simulink subsystem "VehicleBody6DOFSSC"  (R2024a)
settings: Solver=VariableStepAuto  StartTime=0.0  StopTime=10.0  RelTol=1e-3
undefined symbols (not defined in the file): BdyFrm, EnvAirDen, InertFrm, PlntVehAeroDragCff, PlntVehAeroFrntArea, PlntVehAeroLiftCff, PlntVehCGHgtAxl, PlntVehDstCGFrntAxl, PlntVehDstCGRearAxl, PlntVehInitLatPos, PlntVehInitVertPos, PlntVehMass, PlntVehMultiBody, PlntVehPitchMomentInertia, PlntVehRollMomentInertia, PlntVehYawMomentInertia, X, Y, Z
libraries: sm_lib x44, nesl_utility x44, sharedtransform x12, fl_lib x4, vehdynlibeomcommon x3, matrix_library x1
(part 2 of 2)

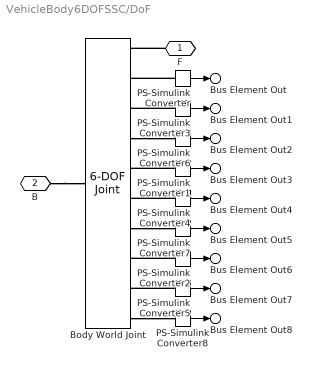
== system VehicleBody6DOFSSC/DoF ==
  Body World Joint : sm_lib/Joints/6-DOF Joint  JointMode=Normal  CompositeWrenchDir=FollowerOnBase  CompositeWrenchFrame=BaseFrame  SenseConstraintForce=off  SenseConstraintTorque=off  SenseTotalForce=off  SenseTotalTorque=off  PxPositionTargetSpecify=on  PxPositionTargetPriority=Low  PxPositionTargetValue=PlntVehInitLongPos  PxPositionTargetValueUnits=m  PxVelocityTargetSpecify=on  PxVelocityTargetPriority=Low  PxVelocityTargetValue=0  PxVelocityTargetValueUnits=m/s  PxEquilibriumPosition=0  PxEquilibriumPositionUnits=m  PxSpringStiffness=0  PxSpringStiffnessUnits=N/m  PxDampingCoefficient=0  PxDampingCoefficientUnits=N/(m/s)  PxLowerLimitSpecify=off  PxLowerLimitBound=-1  PxLowerLimitBoundUnits=m  PxLowerLimitStiffness=1e6  PxLowerLimitStiffnessUnits=N/m  PxLowerLimitDamping=1e3  PxLowerLimitDampingUnits=N/(m/s)  PxLowerLimitTransitionRegionWidth=1e-4  PxLowerLimitTransitionRegionWidthUnits=m  PxUpperLimitSpecify=off  PxUpperLimitBound=1  PxUpperLimitBoundUnits=m  PxUpperLimitStiffness=1e6  PxUpperLimitStiffnessUnits=N/m  PxUpperLimitDamping=1e3  PxUpperLimitDampingUnits=N/(m/s)  PxUpperLimitTransitionRegionWidth=1e-4  PxUpperLimitTransitionRegionWidthUnits=m  PxTorqueActuationMode=NoTorque  PxMotionActuationMode=ComputedMotion  PxSensePosition=on  PxSenseVelocity=on  PxSenseAcceleration=on  PxSenseTorqueForce=off  PxSenseLowerLimitTorqueForce=off  PxSenseUpperLimitTorqueForce=off  PyPositionTargetSpecify=on  PyPositionTargetPriority=Low  PyPositionTargetValue=-PlntVehInitLatPos  PyPositionTargetValueUnits=m  PyVelocityTargetSpecify=on  PyVelocityTargetPriority=Low  PyVelocityTargetValue=0  PyVelocityTargetValueUnits=m/s  PyEquilibriumPosition=0  PyEquilibriumPositionUnits=m  PySpringStiffness=0  PySpringStiffnessUnits=N/m  PyDampingCoefficient=0  PyDampingCoefficientUnits=N/(m/s)  PyLowerLimitSpecify=off  PyLowerLimitBound=-1  PyLowerLimitBoundUnits=m  PyLowerLimitStiffness=1e6  PyLowerLimitStiffnessUnits=N/m  PyLowerLimitDamping=1e3  PyLowerLimitDampingUnits=N/(m/s)  PyLowerLimitTransitionRegionWidth=1e-4  PyLowerLimitTransitionRegionWidthUnits=m  PyUpperLimitSpecify=off  PyUpperLimitBound=1  PyUpperLimitBoundUnits=m  PyUpperLimitStiffness=1e6  PyUpperLimitStiffnessUnits=N/m  PyUpperLimitDamping=1e3  PyUpperLimitDampingUnits=N/(m/s)  PyUpperLimitTransitionRegionWidth=1e-4  PyUpperLimitTransitionRegionWidthUnits=m  PyTorqueActuationMode=NoTorque  PyMotionActuationMode=ComputedMotion  PySensePosition=on  PySenseVelocity=on  PySenseAcceleration=on  PySenseTorqueForce=off  PySenseLowerLimitTorqueForce=off  PySenseUpperLimitTorqueForce=off  PzPositionTargetSpecify=on  PzPositionTargetPriority=Low  PzPositionTargetValue=-PlntVehInitVertPos*0  PzPositionTargetValueUnits=m  PzVelocityTargetSpecify=on  PzVelocityTargetPriority=Low  PzVelocityTargetValue=0  PzVelocityTargetValueUnits=m/s  PzEquilibriumPosition=0  PzEquilibriumPositionUnits=m  PzSpringStiffness=0  PzSpringStiffnessUnits=N/m  PzDampingCoefficient=0  PzDampingCoefficientUnits=N/(m/s)  PzLowerLimitSpecify=off  PzLowerLimitBound=-1  PzLowerLimitBoundUnits=m  PzLowerLimitStiffness=1e6  PzLowerLimitStiffnessUnits=N/m  PzLowerLimitDamping=1e3  PzLowerLimitDampingUnits=N/(m/s)  PzLowerLimitTransitionRegionWidth=1e-4  PzLowerLimitTransitionRegionWidthUnits=m  PzUpperLimitSpecify=off  PzUpperLimitBound=1  PzUpperLimitBoundUnits=m  PzUpperLimitStiffness=1e6  PzUpperLimitStiffnessUnits=N/m  PzUpperLimitDamping=1e3  PzUpperLimitDampingUnits=N/(m/s)  PzUpperLimitTransitionRegionWidth=1e-4  PzUpperLimitTransitionRegionWidthUnits=m  PzTorqueActuationMode=NoTorque  PzMotionActuationMode=ComputedMotion  PzSensePosition=on  PzSenseVelocity=on  PzSenseAcceleration=on  PzSenseTorqueForce=off  PzSenseLowerLimitTorqueForce=off  PzSenseUpperLimitTorqueForce=off  SphPositionTargetSpecify=on  SphPositionTargetPriority=Low  SphPositionTargetRotationMethod=RotationSequence  SphPositionTargetFollAlignAxisA=+X  SphPositionTargetBaseAlignAxisA=+Y  SphPositionTargetFollAlignAxisB=+Y  SphPositionTargetBaseAlignAxisB=+Z  SphPositionTargetRotationStandardAxis=+Z  SphPositionTargetRotationAngle=0.0  SphPositionTargetRotationAngleUnits=deg  SphPositionTargetRotationArbitraryAxis=[0 0 1]  SphPositionTargetRotationSequenceAxes=BaseAxes  SphPositionTargetRotationSequence=XYZ  SphPositionTargetRotationSequenceAngles=[0 0 0]  SphPositionTargetRotationSequenceAnglesUnits=deg  SphPositionTargetRotationMatrix=[1 0 0; 0 1 0; 0 0 1]  SphPositionTargetQuaternion=[1 0 0 0]  SphVelocityTargetSpecify=off  SphVelocityTargetPriority=High  SphVelocityTargetValue=[0 0 0]  SphVelocityTargetValueUnits=deg/s  SphVelocityTargetInFollowerFrame=on  SphEqPosRotationMethod=None  SphEqPosFollAlignAxisA=+X  SphEqPosBaseAlignAxisA=+Y  SphEqPosFollAlignAxisB=+Y  SphEqPosBaseAlignAxisB=+Z  SphEqPosRotationStandardAxis=+Z  SphEqPosRotationAngle=0.0  SphEqPosRotationAngleUnits=deg  SphEqPosRotationArbitraryAxis=[0 0 1]  SphEqPosRotationSequenceAxes=FollowerAxes  SphEqPosRotationSequence=XYX  SphEqPosRotationSequenceAngles=[0 0 0]  SphEqPosRotationSequenceAnglesUnits=deg  SphEqPosRotationMatrix=[1 0 0; 0 1 0; 0 0 1]  SphEqPosQuaternion=[1 0 0 0]  SphSpringStiffness=0  SphSpringStiffnessUnits=N*m/deg  SphDampingCoefficient=0  SphDampingCoefficientUnits=N*m/(deg/s)  SphLowerLimitSpecify=off  SphLowerLimitBound=15  SphLowerLimitBoundUnits=deg  SphLowerLimitStiffness=1e4  SphLowerLimitStiffnessUnits=N*m/deg  SphLowerLimitDamping=10  SphLowerLimitDampingUnits=N*m/(deg/s)  SphLowerLimitTransitionRegionWidth=0.1  SphLowerLimitTransitionRegionWidthUnits=deg  SphUpperLimitSpecify=off  SphUpperLimitBound=45  SphUpperLimitBoundUnits=deg  SphUpperLimitStiffness=1e4  SphUpperLimitStiffnessUnits=N*m/deg  SphUpperLimitDamping=10  SphUpperLimitDampingUnits=N*m/(deg/s)  SphUpperLimitTransitionRegionWidth=0.1  SphUpperLimitTransitionRegionWidthUnits=deg  SphTorqueActuationMode=NoTorque  SphActuateTorqueX=off  SphActuateTorqueY=off  SphActuateTorqueZ=off  SphActuateTorque=off  SphActuationFrame=BaseFrame  SphSensePosition=off  SphSenseVelocityX=off  SphSenseVelocityY=off  SphSenseVelocityZ=off  SphSenseVelocity=off  SphSenseAccelerationX=off  SphSenseAccelerationY=off  SphSenseAccelerationZ=off  SphSenseAcceleration=off  SphSenseLowerLimitTorqueMag=off  SphSenseUpperLimitTorqueMag=off  SphSensingFrame=BaseFrame
  PS-Simulink Converter : nesl_utility/PS-Simulink Converter  PhysicalDomain=network_engine_domain  SubClassName=ps_output  LeftPortType=input  RightPortType=output  PseudoPeriodic=off  Frequencies=[]  VectorFormat=1-D array  Unit=m  AffineConversion=off
  PS-Simulink Converter1 : nesl_utility/PS-Simulink Converter  PhysicalDomain=network_engine_domain  SubClassName=ps_output  LeftPortType=input  RightPortType=output  PseudoPeriodic=off  Frequencies=[]  VectorFormat=1-D array  Unit=m  AffineConversion=off
  PS-Simulink Converter2 : nesl_utility/PS-Simulink Converter  PhysicalDomain=network_engine_domain  SubClassName=ps_output  LeftPortType=input  RightPortType=output  PseudoPeriodic=off  Frequencies=[]  VectorFormat=1-D array  Unit=m  AffineConversion=off
  PS-Simulink Converter3 : nesl_utility/PS-Simulink Converter  PhysicalDomain=network_engine_domain  SubClassName=ps_output  LeftPortType=input  RightPortType=output  PseudoPeriodic=off  Frequencies=[]  VectorFormat=1-D array  Unit=m/s  AffineConversion=off
  PS-Simulink Converter4 : nesl_utility/PS-Simulink Converter  PhysicalDomain=network_engine_domain  SubClassName=ps_output  LeftPortType=input  RightPortType=output  PseudoPeriodic=off  Frequencies=[]  VectorFormat=1-D array  Unit=m/s  AffineConversion=off
  PS-Simulink Converter5 : nesl_utility/PS-Simulink Converter  PhysicalDomain=network_engine_domain  SubClassName=ps_output  LeftPortType=input  RightPortType=output  PseudoPeriodic=off  Frequencies=[]  VectorFormat=1-D array  Unit=m/s  AffineConversion=off
  PS-Simulink Converter6 : nesl_utility/PS-Simulink Converter  PhysicalDomain=network_engine_domain  SubClassName=ps_output  LeftPortType=input  RightPortType=output  PseudoPeriodic=off  Frequencies=[]  VectorFormat=1-D array  Unit=m/s^2  AffineConversion=off
  PS-Simulink Converter7 : nesl_utility/PS-Simulink Converter  PhysicalDomain=network_engine_domain  SubClassName=ps_output  LeftPortType=input  RightPortType=output  PseudoPeriodic=off  Frequencies=[]  VectorFormat=1-D array  Unit=m/s^2  AffineConversion=off
  PS-Simulink Converter8 : nesl_utility/PS-Simulink Converter  PhysicalDomain=network_engine_domain  SubClassName=ps_output  LeftPortType=input  RightPortType=output  PseudoPeriodic=off  Frequencies=[]  VectorFormat=1-D array  Unit=m/s^2  AffineConversion=off
  F : PMIOPort  Side=Left
  B : PMIOPort  Port=2  Side=Right
  Bus Element Out : Outport  VectorParamsAs1DForOutWhenUnconnected=off  PortName=World  Element=x
  Bus Element Out3 : Outport  VectorParamsAs1DForOutWhenUnconnected=off  PortName=World  Element=y
  Bus Element Out6 : Outport  VectorParamsAs1DForOutWhenUnconnected=off  PortName=World  Element=z
  Bus Element Out1 : Outport  VectorParamsAs1DForOutWhenUnconnected=off  PortName=World  Element=vx
  Bus Element Out4 : Outport  VectorParamsAs1DForOutWhenUnconnected=off  PortName=World  Element=vy
  Bus Element Out7 : Outport  VectorParamsAs1DForOutWhenUnconnected=off  PortName=World  Element=vz
  Bus Element Out2 : Outport  VectorParamsAs1DForOutWhenUnconnected=off  PortName=World  Element=gx
  Bus Element Out5 : Outport  VectorParamsAs1DForOutWhenUnconnected=off  PortName=World  Element=gy
  Bus Element Out8 : Outport  VectorParamsAs1DForOutWhenUnconnected=off  PortName=World  Element=gz
  wires:
  PS-Simulink Converter8/1 -> Bus Element Out8/1
  PS-Simulink Converter7/1 -> Bus Element Out5/1
  PS-Simulink Converter5/1 -> Bus Element Out7/1
  PS-Simulink Converter4/1 -> Bus Element Out4/1
  PS-Simulink Converter3/1 -> Bus Element Out1/1
  PS-Simulink Converter6/1 -> Bus Element Out2/1
  PS-Simulink Converter2/1 -> Bus Element Out6/1
  PS-Simulink Converter/1 -> Bus Element Out/1
  PS-Simulink Converter1/1 -> Bus Element Out3/1
  connections:
  PS-Simulink Converter5/LConn1 -- Body World Joint/RConn9
  Body World Joint/RConn7 -- PS-Simulink Converter7/LConn1
  PS-Simulink Converter1/LConn1 -- Body World Joint/RConn5
  PS-Simulink Converter4/LConn1 -- Body World Joint/RConn6
  PS-Simulink Converter3/LConn1 -- Body World Joint/RConn3
  PS-Simulink Converter/LConn1 -- Body World Joint/RConn2
  B/RConn1 -- Body World Joint/LConn1
  Body World Joint/RConn4 -- PS-Simulink Converter6/LConn1
  Body World Joint/RConn10 -- PS-Simulink Converter8/LConn1
  F/RConn1 -- Body World Joint/RConn1
  PS-Simulink Converter2/LConn1 -- Body World Joint/RConn8

== system VehicleBody6DOFSSC/World ==
  MechanismConfiguration : sm_lib/Utilities/Mechanism Configuration  UniformGravity=Constant  GravityVector=[0 0 -9.80665]  GravityVectorUnits=m/s^2  LinearizationDelta=0.001  JointModeTransitionNonlinearIterations=2
  World Frame : sm_lib/Frames and Transforms/World Frame
  W : PMIOPort  Side=Right
  connections:
  MechanismConfiguration/RConn1 -- W/RConn1 -- World Frame/RConn1

== system VehicleBody6DOFSSC/Body Sensor/Cg ==
  InertFrm : Inport
  Bus Creator4 : BusCreator  Inputs=3
  vehBus_Values_InertFrm_Cg_Ang : Subsystem
  vehBus_Values_InertFrm_Cg_Disp : Subsystem
  vehBus_Values_InertFrm_Cg_Vel : Subsystem
  Out1 : Outport
  wires:
  InertFrm/1 -> vehBus_Values_InertFrm_Cg_Vel/1(In), vehBus_Values_InertFrm_Cg_Disp/1(In), vehBus_Values_InertFrm_Cg_Ang/1(In)
  vehBus_Values_InertFrm_Cg_Disp/1(Out1) -> Bus Creator4/1  "Disp"
  vehBus_Values_InertFrm_Cg_Vel/1(Out1) -> Bus Creator4/2  "Vel"
  vehBus_Values_InertFrm_Cg_Ang/1(Out2) -> Bus Creator4/3  "Ang"
  Bus Creator4/1 -> Out1/1

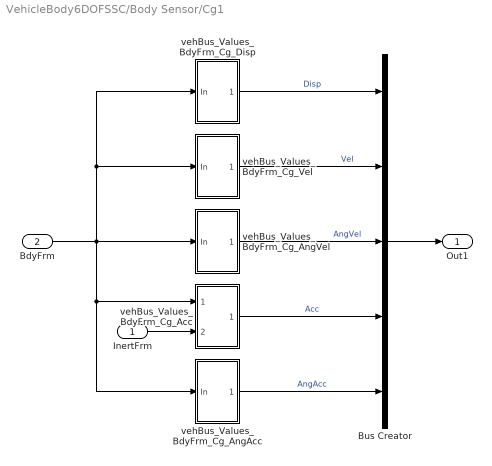
== system VehicleBody6DOFSSC/Body Sensor/Cg1 ==
  InertFrm : Inport
  BdyFrm : Inport  Port=2
  Bus Creator : BusCreator  Inputs=5
  vehBus_Values_BdyFrm_Cg_Acc : Subsystem
  vehBus_Values_BdyFrm_Cg_AngAcc : Subsystem
  vehBus_Values_BdyFrm_Cg_AngVel : Subsystem
  vehBus_Values_BdyFrm_Cg_Disp : Subsystem
  vehBus_Values_BdyFrm_Cg_Vel : Subsystem
  Out1 : Outport
  wires:
  vehBus_Values_BdyFrm_Cg_Vel/1(Out1) -> Bus Creator/2  "Vel"
  vehBus_Values_BdyFrm_Cg_AngVel/1(Out2) -> Bus Creator/3  "AngVel"
  vehBus_Values_BdyFrm_Cg_Acc/1(Out2) -> Bus Creator/4  "Acc"
  Bus Creator/1 -> Out1/1
  BdyFrm/1 -> vehBus_Values_BdyFrm_Cg_AngVel/1(In), vehBus_Values_BdyFrm_Cg_Acc/1(BdyFrm), vehBus_Values_BdyFrm_Cg_AngAcc/1(In), vehBus_Values_BdyFrm_Cg_Vel/1(In), vehBus_Values_BdyFrm_Cg_Disp/1(In)
  InertFrm/1 -> vehBus_Values_BdyFrm_Cg_Acc/2(InertFrm)
  vehBus_Values_BdyFrm_Cg_Disp/1(Out2) -> Bus Creator/1  "Disp"
  vehBus_Values_BdyFrm_Cg_AngAcc/1(Out2) -> Bus Creator/5  "AngAcc"

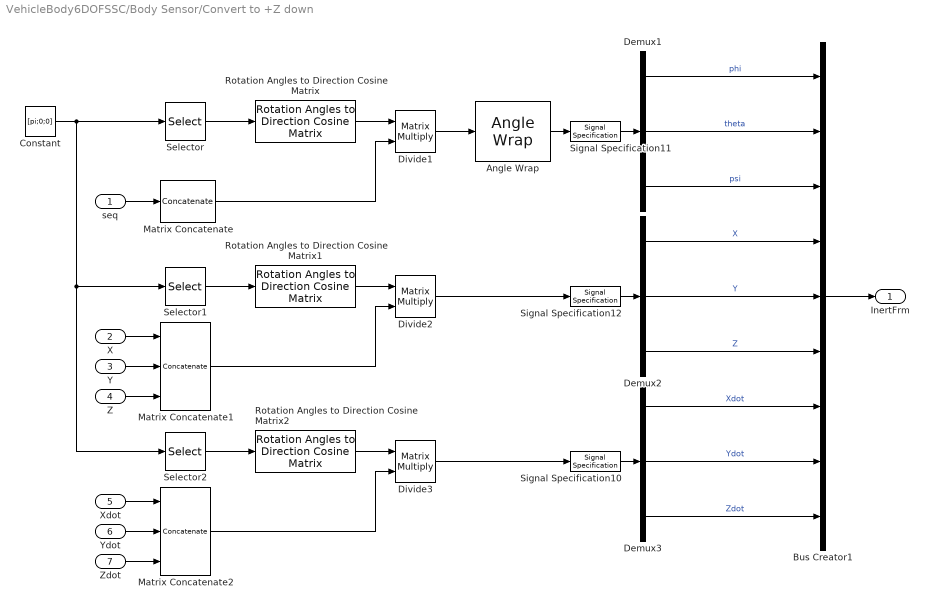
== system VehicleBody6DOFSSC/Body Sensor/Convert to +Z down ==
  seq : Inport
  X : Inport  Port=2
  Y : Inport  Port=3
  Z : Inport  Port=4
  Xdot : Inport  Port=5
  Ydot : Inport  Port=6
  Zdot : Inport  Port=7
  Angle Wrap : vehdynlibeomcommon/6 DOF Generic Vehicle Body/SignalCollection/Angle Wrap  SystemSampleTime=-1  VariantControl=Variant1  LabelModeActiveChoice=Unwrap  VariantActivationTime=update diagram  AllowFlexibleInterface=on  Latency=0  AutoFrameSizeCalculation=off
      link override Unwrap/Unwrap: aMode=6
  Bus Creator1 : BusCreator  Inputs=9
  Constant : Constant  Value=[pi;0;0]  SampleTime=-1
  Demux1 : Demux  Outputs=3
  Demux2 : Demux  Outputs=3
  Demux3 : Demux  Outputs=3
  Divide1 : Product  Inputs=**  Multiplication=Matrix(*)
  Divide2 : Product  Inputs=**  Multiplication=Matrix(*)
  Divide3 : Product  Inputs=**  Multiplication=Matrix(*)
  Matrix Concatenate : Concatenate  NumInputs=1  Mode=Multidimensional array
  Matrix Concatenate1 : Concatenate  NumInputs=3  Mode=Multidimensional array
  Matrix Concatenate2 : Concatenate  NumInputs=3  Mode=Multidimensional array
  Rotation Angles to Direction Cosine Matrix : sharedtransform/Rotation Angles to Direction Cosine Matrix  rotationOrder=ZYX  aMode=2
  Rotation Angles to Direction Cosine Matrix1 : sharedtransform/Rotation Angles to Direction Cosine Matrix  rotationOrder=ZYX  aMode=2
  Rotation Angles to Direction Cosine Matrix2 : sharedtransform/Rotation Angles to Direction Cosine Matrix  rotationOrder=ZYX  aMode=2
  Selector : Selector  InputPortWidth=3  IndexOptions=Index vector (dialog)  Indices=[3 2 1]  OutputSizes=1
  Selector1 : Selector  InputPortWidth=3  IndexOptions=Index vector (dialog)  Indices=[3 2 1]  OutputSizes=1
  Selector2 : Selector  InputPortWidth=3  IndexOptions=Index vector (dialog)  Indices=[3 2 1]  OutputSizes=1
  Signal Specification10 : SignalSpecification  Unit=m/s
  Signal Specification11 : SignalSpecification  Unit=rad
  Signal Specification12 : SignalSpecification  Unit=m
  InertFrm : Outport
  wires:
  Selector/1 -> Rotation Angles to Direction Cosine Matrix/1
  Rotation Angles to Direction Cosine Matrix/1 -> Divide1/1
  Divide1/1 -> Angle Wrap/1
  Demux2/2 -> Bus Creator1/5  "Y"
  Demux3/3 -> Bus Creator1/9  "Zdot"
  Demux1/2 -> Bus Creator1/2  "theta"
  Demux2/3 -> Bus Creator1/6  "Z"
  Demux3/2 -> Bus Creator1/8  "Ydot"
  Demux3/1 -> Bus Creator1/7  "Xdot"
  Demux2/1 -> Bus Creator1/4  "X"
  Demux1/1 -> Bus Creator1/1  "phi"
  Demux1/3 -> Bus Creator1/3  "psi"
  seq/1 -> Matrix Concatenate/1
  Matrix Concatenate/1 -> Divide1/2
  Matrix Concatenate1/1 -> Divide2/2
  X/1 -> Matrix Concatenate1/1
  Rotation Angles to Direction Cosine Matrix1/1 -> Divide2/1
  Selector1/1 -> Rotation Angles to Direction Cosine Matrix1/1
  Divide2/1 -> Signal Specification12/1
  Y/1 -> Matrix Concatenate1/2
  Z/1 -> Matrix Concatenate1/3
  Zdot/1 -> Matrix Concatenate2/3
  Ydot/1 -> Matrix Concatenate2/2
  Selector2/1 -> Rotation Angles to Direction Cosine Matrix2/1
  Rotation Angles to Direction Cosine Matrix2/1 -> Divide3/1
  Constant/1 -> Selector2/1, Selector1/1, Selector/1
  Xdot/1 -> Matrix Concatenate2/1
  Matrix Concatenate2/1 -> Divide3/2
  Divide3/1 -> Signal Specification10/1
  Bus Creator1/1 -> InertFrm/1
  Angle Wrap/1 -> Signal Specification11/1
  Signal Specification10/1 -> Demux3/1
  Signal Specification11/1 -> Demux1/1
  Signal Specification12/1 -> Demux2/1

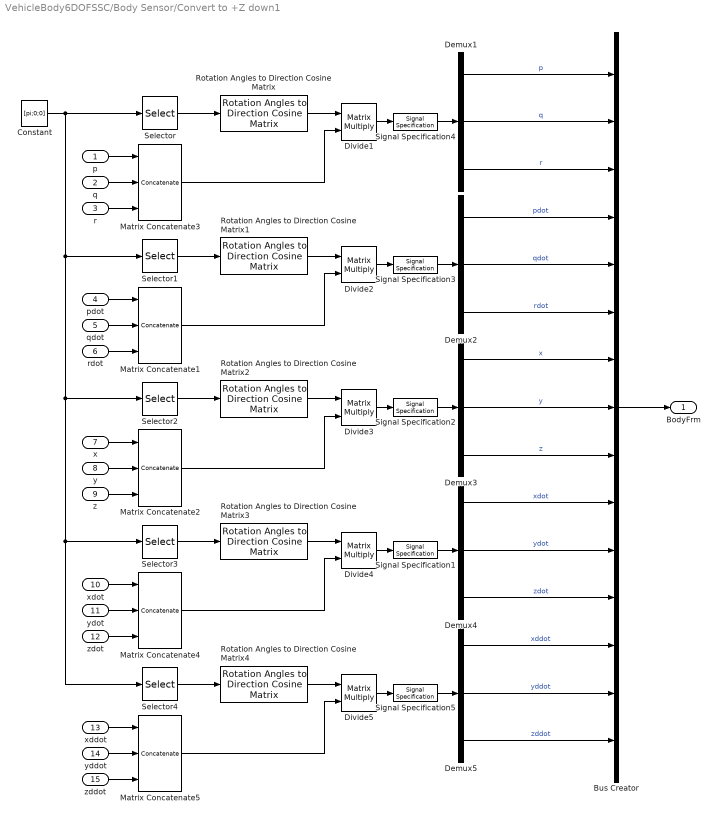
== system VehicleBody6DOFSSC/Body Sensor/Convert to +Z down1 ==
  p : Inport
  q : Inport  Port=2
  r : Inport  Port=3
  pdot : Inport  Port=4
  qdot : Inport  Port=5
  rdot : Inport  Port=6
  x : Inport  Port=7
  y : Inport  Port=8
  z : Inport  Port=9
  xdot : Inport  Port=10
  ydot : Inport  Port=11
  zdot : Inport  Port=12
  xddot : Inport  Port=13
  yddot : Inport  Port=14
  zddot : Inport  Port=15
  Bus Creator : BusCreator  Inputs=15
  Constant : Constant  Value=[pi;0;0]  SampleTime=-1
  Demux{1..5} (5 alike) : Demux  Outputs=3
  Divide{1..5} (5 alike) : Product  Inputs=**  Multiplication=Matrix(*)
  Matrix Concatenate{1..5} (5 alike) : Concatenate  NumInputs=3  Mode=Multidimensional array
  Rotation Angles to Direction Cosine Matrix{,1..4} (5 alike) : sharedtransform/Rotation Angles to Direction Cosine Matrix  rotationOrder=ZYX  aMode=2
  Selector{,1..4} (5 alike) : Selector  InputPortWidth=3  IndexOptions=Index vector (dialog)  Indices=[3 2 1]  OutputSizes=1
  Signal Specification1 : SignalSpecification  Unit=m/s
  Signal Specification2 : SignalSpecification  Unit=m
  Signal Specification3 : SignalSpecification  Unit=rad/s^2
  Signal Specification4 : SignalSpecification  Unit=rad/s
  Signal Specification5 : SignalSpecification  Unit=m/s^2
  BodyFrm : Outport
  wires:
  Divide3/1 -> Signal Specification2/1
  Matrix Concatenate2/1 -> Divide3/2
  x/1 -> Matrix Concatenate2/1
  Rotation Angles to Direction Cosine Matrix2/1 -> Divide3/1
  Selector2/1 -> Rotation Angles to Direction Cosine Matrix2/1
  y/1 -> Matrix Concatenate2/2
  z/1 -> Matrix Concatenate2/3
  rdot/1 -> Matrix Concatenate1/3
  qdot/1 -> Matrix Concatenate1/2
  Divide2/1 -> Signal Specification3/1
  Selector1/1 -> Rotation Angles to Direction Cosine Matrix1/1
  Rotation Angles to Direction Cosine Matrix1/1 -> Divide2/1
  pdot/1 -> Matrix Concatenate1/1
  Matrix Concatenate1/1 -> Divide2/2
  Divide1/1 -> Signal Specification4/1
  Rotation Angles to Direction Cosine Matrix/1 -> Divide1/1
  Selector/1 -> Rotation Angles to Direction Cosine Matrix/1
  Bus Creator/1 -> BodyFrm/1
  Demux1/1 -> Bus Creator/1  "p"
  Demux1/2 -> Bus Creator/2  "q"
  Demux1/3 -> Bus Creator/3  "r"
  Demux2/1 -> Bus Creator/4  "pdot"
  Demux2/2 -> Bus Creator/5  "qdot"
  Demux2/3 -> Bus Creator/6  "rdot"
  Demux3/1 -> Bus Creator/7  "x"
  Demux3/2 -> Bus Creator/8  "y"
  Demux3/3 -> Bus Creator/9  "z"
  Demux4/1 -> Bus Creator/10  "xdot"
  Demux4/2 -> Bus Creator/11  "ydot"
  Demux4/3 -> Bus Creator/12  "zdot"
  Demux5/1 -> Bus Creator/13  "xddot"
  Demux5/2 -> Bus Creator/14  "yddot"
  Demux5/3 -> Bus Creator/15  "zddot"
  Matrix Concatenate3/1 -> Divide1/2
  p/1 -> Matrix Concatenate3/1
  r/1 -> Matrix Concatenate3/3
  q/1 -> Matrix Concatenate3/2
  zdot/1 -> Matrix Concatenate4/3
  ydot/1 -> Matrix Concatenate4/2
  Selector3/1 -> Rotation Angles to Direction Cosine Matrix3/1
  Rotation Angles to Direction Cosine Matrix3/1 -> Divide4/1
  xdot/1 -> Matrix Concatenate4/1
  Matrix Concatenate4/1 -> Divide4/2
  Divide4/1 -> Signal Specification1/1
  Matrix Concatenate5/1 -> Divide5/2
  xddot/1 -> Matrix Concatenate5/1
  Constant/1 -> Selector/1, Selector1/1, Selector4/1, Selector3/1, Selector2/1
  Rotation Angles to Direction Cosine Matrix4/1 -> Divide5/1
  Selector4/1 -> Rotation Angles to Direction Cosine Matrix4/1
  yddot/1 -> Matrix Concatenate5/2
  zddot/1 -> Matrix Concatenate5/3
  Divide5/1 -> Signal Specification5/1
  Signal Specification5/1 -> Demux5/1
  Signal Specification1/1 -> Demux4/1
  Signal Specification2/1 -> Demux3/1
  Signal Specification3/1 -> Demux2/1
  Signal Specification4/1 -> Demux1/1

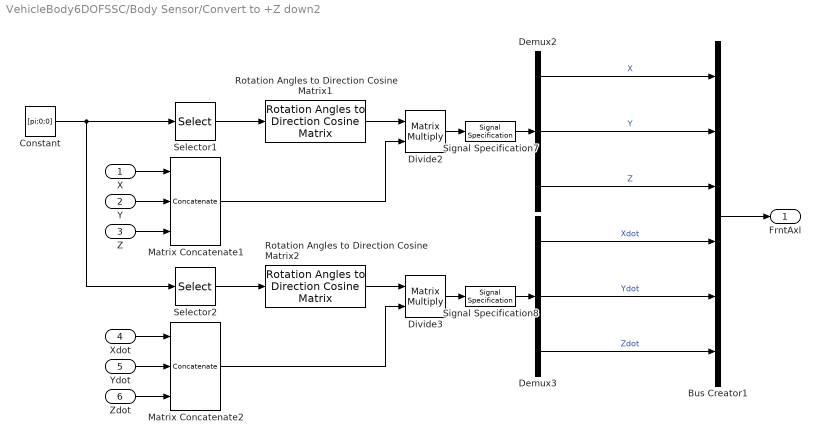
== system VehicleBody6DOFSSC/Body Sensor/Convert to +Z down2 ==
  X : Inport
  Y : Inport  Port=2
  Z : Inport  Port=3
  Xdot : Inport  Port=4
  Ydot : Inport  Port=5
  Zdot : Inport  Port=6
  Bus Creator1 : BusCreator  Inputs=6
  Constant : Constant  Value=[pi;0;0]  SampleTime=-1
  Demux2 : Demux  Outputs=3
  Demux3 : Demux  Outputs=3
  Divide2 : Product  Inputs=**  Multiplication=Matrix(*)
  Divide3 : Product  Inputs=**  Multiplication=Matrix(*)
  Matrix Concatenate1 : Concatenate  NumInputs=3  Mode=Multidimensional array
  Matrix Concatenate2 : Concatenate  NumInputs=3  Mode=Multidimensional array
  Rotation Angles to Direction Cosine Matrix1 : sharedtransform/Rotation Angles to Direction Cosine Matrix  rotationOrder=ZYX  aMode=2
  Rotation Angles to Direction Cosine Matrix2 : sharedtransform/Rotation Angles to Direction Cosine Matrix  rotationOrder=ZYX  aMode=2
  Selector1 : Selector  InputPortWidth=3  IndexOptions=Index vector (dialog)  Indices=[3 2 1]  OutputSizes=1
  Selector2 : Selector  InputPortWidth=3  IndexOptions=Index vector (dialog)  Indices=[3 2 1]  OutputSizes=1
  Signal Specification7 : SignalSpecification  Unit=m
  Signal Specification8 : SignalSpecification  Unit=m/s
  FrntAxl : Outport
  wires:
  Bus Creator1/1 -> FrntAxl/1
  Divide3/1 -> Signal Specification8/1
  Matrix Concatenate2/1 -> Divide3/2
  Xdot/1 -> Matrix Concatenate2/1
  Constant/1 -> Selector1/1, Selector2/1
  Rotation Angles to Direction Cosine Matrix2/1 -> Divide3/1
  Selector2/1 -> Rotation Angles to Direction Cosine Matrix2/1
  Ydot/1 -> Matrix Concatenate2/2
  Zdot/1 -> Matrix Concatenate2/3
  Z/1 -> Matrix Concatenate1/3
  Y/1 -> Matrix Concatenate1/2
  Divide2/1 -> Signal Specification7/1
  Selector1/1 -> Rotation Angles to Direction Cosine Matrix1/1
  Rotation Angles to Direction Cosine Matrix1/1 -> Divide2/1
  X/1 -> Matrix Concatenate1/1
  Matrix Concatenate1/1 -> Divide2/2
  Demux2/1 -> Bus Creator1/1  "X"
  Demux3/1 -> Bus Creator1/4  "Xdot"
  Demux3/2 -> Bus Creator1/5  "Ydot"
  Demux2/3 -> Bus Creator1/3  "Z"
  Demux3/3 -> Bus Creator1/6  "Zdot"
  Demux2/2 -> Bus Creator1/2  "Y"
  Signal Specification7/1 -> Demux2/1
  Signal Specification8/1 -> Demux3/1

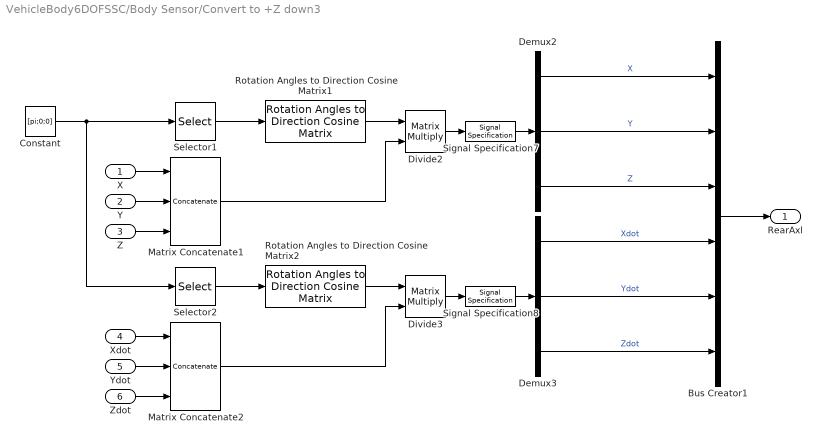
== system VehicleBody6DOFSSC/Body Sensor/Convert to +Z down3 ==
  X : Inport
  Y : Inport  Port=2
  Z : Inport  Port=3
  Xdot : Inport  Port=4
  Ydot : Inport  Port=5
  Zdot : Inport  Port=6
  Bus Creator1 : BusCreator  Inputs=6
  Constant : Constant  Value=[pi;0;0]  SampleTime=-1
  Demux2 : Demux  Outputs=3
  Demux3 : Demux  Outputs=3
  Divide2 : Product  Inputs=**  Multiplication=Matrix(*)
  Divide3 : Product  Inputs=**  Multiplication=Matrix(*)
  Matrix Concatenate1 : Concatenate  NumInputs=3  Mode=Multidimensional array
  Matrix Concatenate2 : Concatenate  NumInputs=3  Mode=Multidimensional array
  Rotation Angles to Direction Cosine Matrix1 : sharedtransform/Rotation Angles to Direction Cosine Matrix  rotationOrder=ZYX  aMode=2
  Rotation Angles to Direction Cosine Matrix2 : sharedtransform/Rotation Angles to Direction Cosine Matrix  rotationOrder=ZYX  aMode=2
  Selector1 : Selector  InputPortWidth=3  IndexOptions=Index vector (dialog)  Indices=[3 2 1]  OutputSizes=1
  Selector2 : Selector  InputPortWidth=3  IndexOptions=Index vector (dialog)  Indices=[3 2 1]  OutputSizes=1
  Signal Specification7 : SignalSpecification  Unit=m
  Signal Specification8 : SignalSpecification  Unit=m/s
  RearAxl : Outport
  wires:
  Demux2/2 -> Bus Creator1/2  "Y"
  Demux3/3 -> Bus Creator1/6  "Zdot"
  Demux2/3 -> Bus Creator1/3  "Z"
  Demux3/2 -> Bus Creator1/5  "Ydot"
  Demux3/1 -> Bus Creator1/4  "Xdot"
  Demux2/1 -> Bus Creator1/1  "X"
  Matrix Concatenate1/1 -> Divide2/2
  X/1 -> Matrix Concatenate1/1
  Rotation Angles to Direction Cosine Matrix1/1 -> Divide2/1
  Selector1/1 -> Rotation Angles to Direction Cosine Matrix1/1
  Divide2/1 -> Signal Specification7/1
  Y/1 -> Matrix Concatenate1/2
  Z/1 -> Matrix Concatenate1/3
  Zdot/1 -> Matrix Concatenate2/3
  Ydot/1 -> Matrix Concatenate2/2
  Selector2/1 -> Rotation Angles to Direction Cosine Matrix2/1
  Rotation Angles to Direction Cosine Matrix2/1 -> Divide3/1
  Constant/1 -> Selector2/1, Selector1/1
  Xdot/1 -> Matrix Concatenate2/1
  Matrix Concatenate2/1 -> Divide3/2
  Divide3/1 -> Signal Specification8/1
  Bus Creator1/1 -> RearAxl/1
  Signal Specification7/1 -> Demux2/1
  Signal Specification8/1 -> Demux3/1

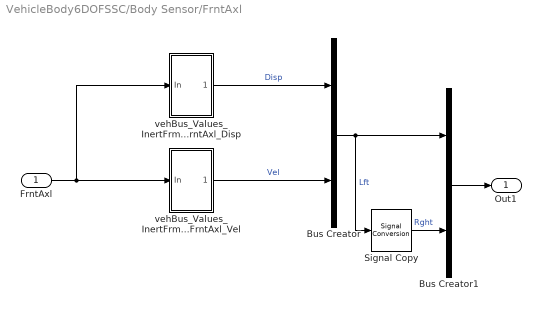
== system VehicleBody6DOFSSC/Body Sensor/FrntAxl ==
  FrntAxl : Inport
  Bus Creator : BusCreator  Inputs=2
  Bus Creator1 : BusCreator  Inputs=2
  Signal Copy : SignalConversion  OverrideOpt=off
  vehBus_Values_InertFrm_FrntAxl_Disp : Subsystem
  vehBus_Values_InertFrm_FrntAxl_Vel : Subsystem
  Out1 : Outport
  wires:
  Bus Creator1/1 -> Out1/1
  Signal Copy/1 -> Bus Creator1/2  "Rght"
  vehBus_Values_InertFrm_FrntAxl_Disp/1(Out1) -> Bus Creator/1  "Disp"
  vehBus_Values_InertFrm_FrntAxl_Vel/1(Out1) -> Bus Creator/2  "Vel"
  Bus Creator/1 -> Bus Creator1/1, Signal Copy/1  "Lft"
  FrntAxl/1 -> vehBus_Values_InertFrm_FrntAxl_Disp/1(In), vehBus_Values_InertFrm_FrntAxl_Vel/1(In)

== system VehicleBody6DOFSSC/Body Sensor/Geom ==
  note: Assumes no Geometric
      | Simulation offsets
  InertFrm : Inport
  Bus Creator3 : BusCreator  Inputs=2
  vehBus_Values_InertFrm_Geom_Disp : Subsystem
  vehBus_Values_InertFrm_Geom_Vel : Subsystem
  Out1 : Outport
  wires:
  Bus Creator3/1 -> Out1/1
  vehBus_Values_InertFrm_Geom_Vel/1(Out1) -> Bus Creator3/2  "Vel"
  vehBus_Values_InertFrm_Geom_Disp/1(Out1) -> Bus Creator3/1  "Disp"
  InertFrm/1 -> vehBus_Values_InertFrm_Geom_Vel/1(In), vehBus_Values_InertFrm_Geom_Disp/1(In)

== system VehicleBody6DOFSSC/Body Sensor/RearAxl ==
  RearAxl1 : Inport
  Bus Creator1 : BusCreator  Inputs=2
  Bus Creator2 : BusCreator  Inputs=2
  Signal Copy : SignalConversion  OverrideOpt=off
  vehBus_Values_InertFrm_RearAxl_Disp : Subsystem
  vehBus_Values_InertFrm_RearAxl_Vel : Subsystem
  Out1 : Outport
  wires:
  Bus Creator2/1 -> Out1/1
  Signal Copy/1 -> Bus Creator2/2  "Rght"
  Bus Creator1/1 -> Bus Creator2/1, Signal Copy/1  "Lft"
  vehBus_Values_InertFrm_RearAxl_Disp/1(Out1) -> Bus Creator1/1  "Disp"
  vehBus_Values_InertFrm_RearAxl_Vel/1(Out1) -> Bus Creator1/2  "Vel"
  RearAxl1/1 -> vehBus_Values_InertFrm_RearAxl_Disp/1(In), vehBus_Values_InertFrm_RearAxl_Vel/1(In)

== system VehicleBody6DOFSSC/Body Sensor/Cg/vehBus_Values_InertFrm_Cg_Ang ==
  In : Inport
  Bus Selector : BusSelector  OutputSignals=phi,theta,psi
  busOut1 : BusCreator  Inputs=3
  Out2 : Outport
  wires:
  busOut1/1 -> Out2/1
  Bus Selector/3 -> busOut1/3  "<psi>"
  Bus Selector/2 -> busOut1/2  "<theta>"
  In/1 -> Bus Selector/1
  Bus Selector/1 -> busOut1/1  "<phi>"

== system VehicleBody6DOFSSC/Body Sensor/Cg/vehBus_Values_InertFrm_Cg_Disp ==
  In : Inport
  Bus Selector : BusSelector  OutputSignals=X,Y,Z
  busOut : BusCreator  Inputs=3
  Out1 : Outport
  wires:
  busOut/1 -> Out1/1
  In/1 -> Bus Selector/1
  Bus Selector/1 -> busOut/1  "<X>"
  Bus Selector/2 -> busOut/2  "<Y>"
  Bus Selector/3 -> busOut/3  "<Z>"

== system VehicleBody6DOFSSC/Body Sensor/Cg/vehBus_Values_InertFrm_Cg_Vel ==
  In : Inport
  Bus Selector : BusSelector  OutputSignals=Xdot,Ydot,Zdot
  busOut : BusCreator  Inputs=3
  Out1 : Outport
  wires:
  busOut/1 -> Out1/1
  In/1 -> Bus Selector/1
  Bus Selector/1 -> busOut/1  "<Xdot>"
  Bus Selector/2 -> busOut/2  "<Ydot>"
  Bus Selector/3 -> busOut/3  "<Zdot>"

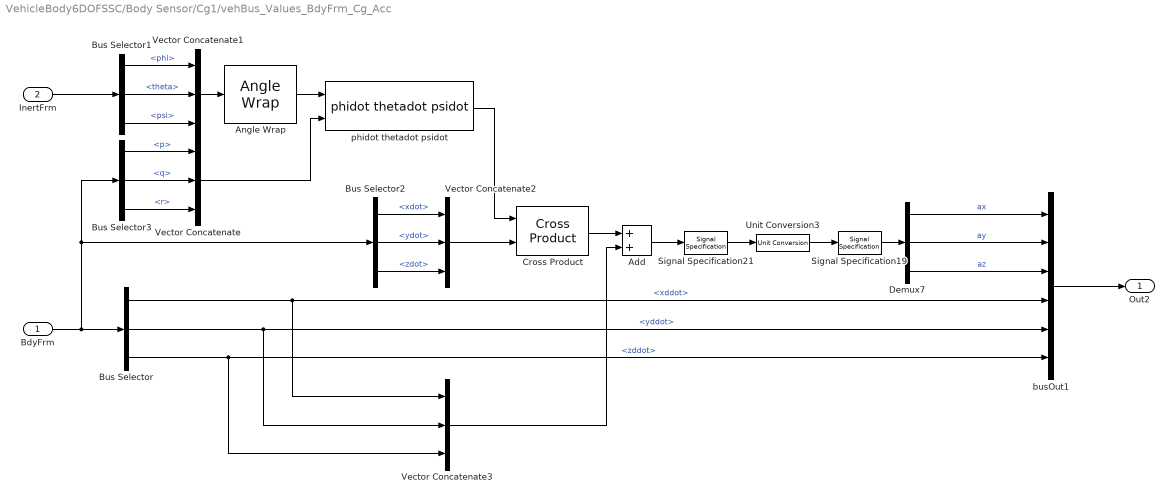
== system VehicleBody6DOFSSC/Body Sensor/Cg1/vehBus_Values_BdyFrm_Cg_Acc ==
  BdyFrm : Inport
  InertFrm : Inport  Port=2
  Add : Sum
  Angle Wrap : vehdynlibeomcommon/6 DOF Generic Vehicle Body/SignalCollection/Angle Wrap  SystemSampleTime=-1  VariantControl=Variant1  LabelModeActiveChoice=Unwrap  VariantActivationTime=update diagram  AllowFlexibleInterface=on  Latency=0  AutoFrameSizeCalculation=off
      link override Unwrap/Unwrap: aMode=6
  Bus Selector : BusSelector  OutputSignals=xddot,yddot,zddot
  Bus Selector1 : BusSelector  OutputSignals=phi,theta,psi
  Bus Selector2 : BusSelector  OutputSignals=xdot,ydot,zdot
  Bus Selector3 : BusSelector  OutputSignals=p,q,r
  Cross Product : matrix_library/Cross Product
  Demux7 : Demux  Outputs=3
  Signal Specification19 : SignalSpecification  Unit=gn
  Signal Specification21 : SignalSpecification  Unit=m/s^2
  Unit Conversion3 : UnitConversion
  Vector Concatenate{,1..3} (4 alike) : Concatenate  NumInputs=3
  busOut1 : BusCreator  Inputs=6
  phidot thetadot psidot : vehdynlibeomcommon/6 DOF Generic Vehicle Body/SignalCollection/phidot thetadot psidot  SystemSampleTime=-1  VariantActivationTime=update diagram  AllowFlexibleInterface=on  Latency=0  AutoFrameSizeCalculation=off
  Out2 : Outport
  wires:
  busOut1/1 -> Out2/1
  Bus Selector/3 -> busOut1/6, Vector Concatenate3/3  "<zddot>"
  Bus Selector/2 -> busOut1/5, Vector Concatenate3/2  "<yddot>"
  BdyFrm/1 -> Bus Selector/1, Bus Selector2/1, Bus Selector3/1
  Bus Selector/1 -> busOut1/4, Vector Concatenate3/1  "<xddot>"
  Vector Concatenate1/1 -> Angle Wrap/1
  Vector Concatenate/1 -> phidot thetadot psidot/2
  Angle Wrap/1 -> phidot thetadot psidot/1
  InertFrm/1 -> Bus Selector1/1
  Bus Selector3/1 -> Vector Concatenate/1  "<p>"
  Bus Selector3/2 -> Vector Concatenate/2  "<q>"
  Bus Selector3/3 -> Vector Concatenate/3  "<r>"
  Bus Selector1/3 -> Vector Concatenate1/3  "<psi>"
  Bus Selector1/2 -> Vector Concatenate1/2  "<theta>"
  Bus Selector1/1 -> Vector Concatenate1/1  "<phi>"
  phidot thetadot psidot/1 -> Cross Product/1
  Bus Selector2/1 -> Vector Concatenate2/1  "<xdot>"
  Bus Selector2/2 -> Vector Concatenate2/2  "<ydot>"
  Bus Selector2/3 -> Vector Concatenate2/3  "<zdot>"
  Vector Concatenate2/1 -> Cross Product/2
  Signal Specification21/1 -> Unit Conversion3/1
  Add/1 -> Signal Specification21/1
  Cross Product/1 -> Add/1
  Vector Concatenate3/1 -> Add/2
  Demux7/1 -> busOut1/1  "ax"
  Unit Conversion3/1 -> Signal Specification19/1
  Demux7/2 -> busOut1/2  "ay"
  Demux7/3 -> busOut1/3  "az"
  Signal Specification19/1 -> Demux7/1

== system VehicleBody6DOFSSC/Body Sensor/Cg1/vehBus_Values_BdyFrm_Cg_AngAcc ==
  In : Inport
  Bus Selector : BusSelector  OutputSignals=pdot,qdot,rdot
  busOut1 : BusCreator  Inputs=3
  Out2 : Outport
  wires:
  busOut1/1 -> Out2/1
  Bus Selector/3 -> busOut1/3  "<rdot>"
  Bus Selector/2 -> busOut1/2  "<qdot>"
  In/1 -> Bus Selector/1
  Bus Selector/1 -> busOut1/1  "<pdot>"

== system VehicleBody6DOFSSC/Body Sensor/Cg1/vehBus_Values_BdyFrm_Cg_AngVel ==
  In : Inport
  Bus Selector : BusSelector  OutputSignals=p,q,r
  busOut1 : BusCreator  Inputs=3
  Out2 : Outport
  wires:
  busOut1/1 -> Out2/1
  Bus Selector/3 -> busOut1/3  "<r>"
  Bus Selector/2 -> busOut1/2  "<q>"
  In/1 -> Bus Selector/1
  Bus Selector/1 -> busOut1/1  "<p>"

== system VehicleBody6DOFSSC/Body Sensor/Cg1/vehBus_Values_BdyFrm_Cg_Disp ==
  In : Inport
  Bus Selector : BusSelector  OutputSignals=x,y,z
  busOut1 : BusCreator  Inputs=3
  Out2 : Outport
  wires:
  busOut1/1 -> Out2/1
  Bus Selector/3 -> busOut1/3  "<z>"
  Bus Selector/2 -> busOut1/2  "<y>"
  In/1 -> Bus Selector/1
  Bus Selector/1 -> busOut1/1  "<x>"

== system VehicleBody6DOFSSC/Body Sensor/Cg1/vehBus_Values_BdyFrm_Cg_Vel ==
  In : Inport
  Bus Selector : BusSelector  OutputSignals=xdot,ydot,zdot
  busOut : BusCreator  Inputs=3
  Out1 : Outport
  wires:
  Bus Selector/3 -> busOut/3  "<zdot>"
  Bus Selector/2 -> busOut/2  "<ydot>"
  Bus Selector/1 -> busOut/1  "<xdot>"
  In/1 -> Bus Selector/1
  busOut/1 -> Out1/1

== system VehicleBody6DOFSSC/Body Sensor/FrntAxl/vehBus_Values_InertFrm_FrntAxl_Disp ==
  In : Inport
  Bus Selector : BusSelector  OutputSignals=X,Y,Z
  busOut : BusCreator  Inputs=3
  Out1 : Outport
  wires:
  busOut/1 -> Out1/1
  Bus Selector/2 -> busOut/2  "<Y>"
  In/1 -> Bus Selector/1
  Bus Selector/3 -> busOut/3  "<Z>"
  Bus Selector/1 -> busOut/1  "<X>"

== system VehicleBody6DOFSSC/Body Sensor/FrntAxl/vehBus_Values_InertFrm_FrntAxl_Vel ==
  In : Inport
  Bus Selector : BusSelector  OutputSignals=Xdot,Ydot,Zdot
  busOut : BusCreator  Inputs=3
  Out1 : Outport
  wires:
  busOut/1 -> Out1/1
  Bus Selector/3 -> busOut/3  "<Zdot>"
  Bus Selector/2 -> busOut/2  "<Ydot>"
  Bus Selector/1 -> busOut/1  "<Xdot>"
  In/1 -> Bus Selector/1

== system VehicleBody6DOFSSC/Body Sensor/Geom/vehBus_Values_InertFrm_Geom_Disp ==
  In : Inport
  Bus Selector : BusSelector  OutputSignals=X,Y,Z
  busOut : BusCreator  Inputs=3
  Out1 : Outport
  wires:
  busOut/1 -> Out1/1
  Bus Selector/1 -> busOut/1  "<X>"
  Bus Selector/3 -> busOut/3  "<Z>"
  In/1 -> Bus Selector/1
  Bus Selector/2 -> busOut/2  "<Y>"

== system VehicleBody6DOFSSC/Body Sensor/Geom/vehBus_Values_InertFrm_Geom_Vel ==
  In : Inport
  Bus Selector : BusSelector  OutputSignals=Xdot,Ydot,Zdot
  busOut : BusCreator  Inputs=3
  Out1 : Outport
  wires:
  busOut/1 -> Out1/1
  Bus Selector/3 -> busOut/3  "<Zdot>"
  Bus Selector/2 -> busOut/2  "<Ydot>"
  Bus Selector/1 -> busOut/1  "<Xdot>"
  In/1 -> Bus Selector/1

== system VehicleBody6DOFSSC/Body Sensor/RearAxl/vehBus_Values_InertFrm_RearAxl_Disp ==
  In : Inport
  Bus Selector : BusSelector  OutputSignals=X,Y,Z
  busOut : BusCreator  Inputs=3
  Out1 : Outport
  wires:
  busOut/1 -> Out1/1
  In/1 -> Bus Selector/1
  Bus Selector/3 -> busOut/3  "<Z>"
  Bus Selector/2 -> busOut/2  "<Y>"
  Bus Selector/1 -> busOut/1  "<X>"

== system VehicleBody6DOFSSC/Body Sensor/RearAxl/vehBus_Values_InertFrm_RearAxl_Vel ==
  In : Inport
  Bus Selector : BusSelector  OutputSignals=Xdot,Ydot,Zdot
  busOut : BusCreator  Inputs=3
  Out1 : Outport
  wires:
  busOut/1 -> Out1/1
  Bus Selector/1 -> busOut/1  "<Xdot>"
  Bus Selector/2 -> busOut/2  "<Ydot>"
  In/1 -> Bus Selector/1
  Bus Selector/3 -> busOut/3  "<Zdot>"
